simulink model "vehicleForcesCalculation"  (R2024b)
settings: Solver=VariableStepAuto  StartTime=0.0  StopTime=10.0  RelTol=1e-3
values from neighbouring files (symbols this model uses):
  air_density = 1.225    [vehicleForcesCalculationValues.m]
  cdrag = 0.3    [vehicleForcesCalculationValues.m]
  frontal_area = 1    [vehicleForcesCalculationValues.m]
  g = 9.8    [vehicleForcesCalculationValues.m]
  mass = 2000    [vehicleForcesCalculationValues.m]
  max_velocity = 120    [vehicleForcesCalculationValues.m]
  theta = 10    [vehicleForcesCalculationValues.m]
  urr = 0.013    [vehicleForcesCalculationValues.m]
undefined symbols (not defined in the file or in its folder): magnitude
libraries: simulink_extras x1

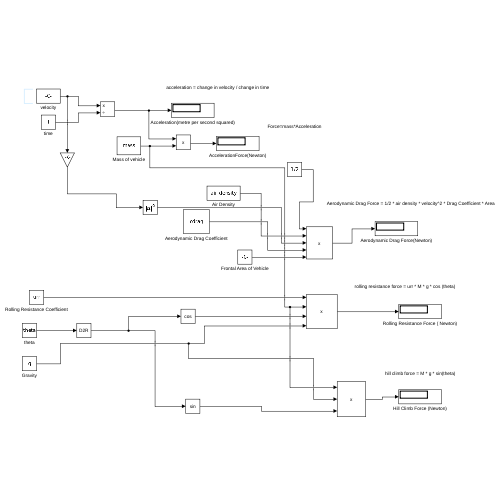
[thumbnail: Simulink's stored preview of the top-level diagram]
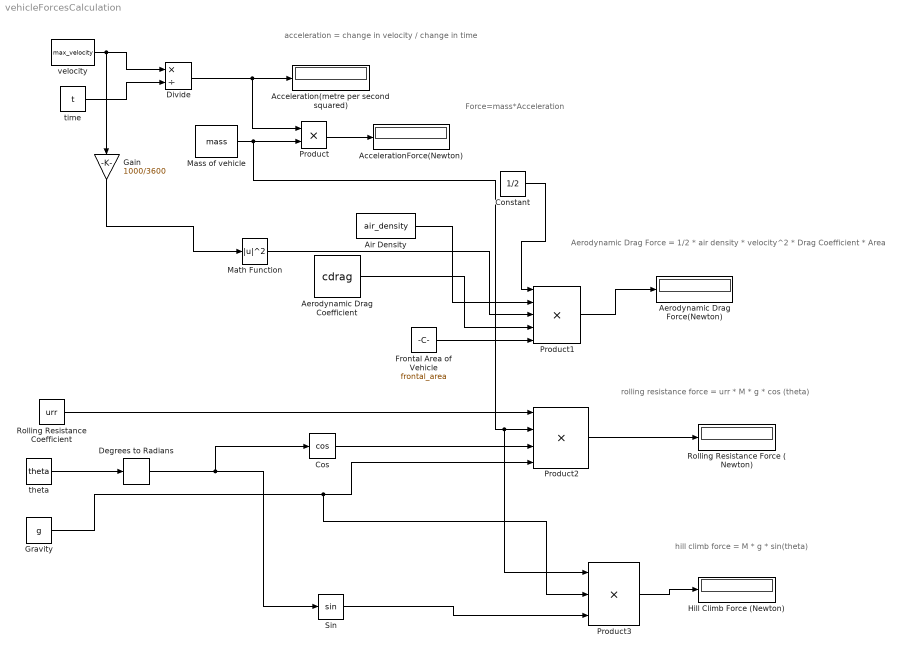
== system vehicleForcesCalculation ==
  note: hill climb force = M * g * sin(theta)
  note: rolling resistance force = urr * M * g * cos (theta)
  note: Aerodynamic Drag Force = 1/2 * air density * velocity^2 * Drag Coefficient * Area
  note: Force=mass*Acceleration
  note: acceleration = change in velocity / change in time
  Acceleration(metre per second squared) : Display
  AccelerationForce(Newton) : Display
  Aerodynamic Drag Coefficient : Constant  Value=cdrag
  Aerodynamic Drag Force(Newton) : Display
  Air Density : Constant  Value=air_density
  Constant : Constant  Value=1/2
  Cos : Trigonometry  Operator=cos
  Degrees to Radians : simulink_extras/Transformations/Degrees to Radians
  Divide : Product  Inputs=*/
  Frontal Area of Vehicle : Constant  Value=frontal_area
  Gain : Gain  Gain=1000/3600
  Gravity : Constant  Value=g
  Hill Climb Force (Newton) : Display
  Mass of vehicle : Constant  Value=mass
  Math Function : Math  Operator=magnitude^2
  Product : Product
  Product1 : Product  Inputs=5
  Product2 : Product  Inputs=4
  Product3 : Product  Inputs=3
  Rolling Resistance Coefficient : Constant  Value=urr
  Rolling Resistance Force ( Newton) : Display
  Sin : Trigonometry
  theta : Constant  Value=theta
  time : Constant  Value=t
  velocity : Constant  Value=max_velocity
  wires:
  velocity/1 -> Divide/1, Gain/1
  time/1 -> Divide/2
  Divide/1 -> Product/1, Acceleration(metre per second squared)/1
  Mass of vehicle/1 -> Product3/1, Product2/2, Product/2
  Product/1 -> AccelerationForce(Newton)/1
  Product1/1 -> Aerodynamic Drag Force(Newton)/1
  Frontal Area of Vehicle/1 -> Product1/5
  Aerodynamic Drag Coefficient/1 -> Product1/4
  Air Density/1 -> Product1/2
  Constant/1 -> Product1/1
  Math Function/1 -> Product1/3
  Gain/1 -> Math Function/1
  Gravity/1 -> Product3/2, Product2/4
  Product2/1 -> Rolling Resistance Force ( Newton)/1
  theta/1 -> Degrees to Radians/1
  Cos/1 -> Product2/3
  Rolling Resistance Coefficient/1 -> Product2/1
  Sin/1 -> Product3/3
  Product3/1 -> Hill Climb Force (Newton)/1
  Degrees to Radians/1 -> Sin/1, Cos/1
